simulink model "autopilot"  (R2020a)
settings: Solver=VariableStepAuto  StartTime=0.0  StopTime=10.0  RelTol=1e-3
values from neighbouring files (symbols this model uses):
  A = [-0.322, 0.052, 0.028, -1.12, 0.002 ... (first row only)    [main.m]
  B = [ (1-t_thr)  X_delta2 ... (first row only)    [Part1.m]    (also in main.m = [0; 0; 0; 0; 7.5;]; part2.m = 21.8; speed_control.m = 21.8)
  C = CRB + CA    [Part1.m]    (also in main.m = [1, 0,0,0,0)
  d = 1.5*pi/180    (= 0.0261799387799)    [main.m]    (also in part2.m = -[Xns Ycf Ncf]'; speed_control.m = -[Xns Ycf Ncf]')
  D = [0; 0; 0; 0;]    [main.m]    (also in part2.m = diag([-Xu -Yv -Nr]); problem4.m = [ Xu 0 0; speed_control.m = diag([-Xu -Yv -Nr]))
  g = 9.81    [main.m]
  kd_phi = (2*zeta_phi*omega_n_phi-a_phi_1)/a_phi_2    [main.m]
  ki_chi = omega_n_chi^2*V_g/g    [main.m]
  ki_phi = 0    [main.m]
  kp_chi = 2*zeta_chi*omega_n_chi*V_g/g    [main.m]
  kp_phi = delta_max/e_max*sign(a_phi_2)    [main.m]
  V_g = 580    [main.m]
libraries: simulink_extras x7
settings Model: Creator=erlended  LastModifiedBy=erlended

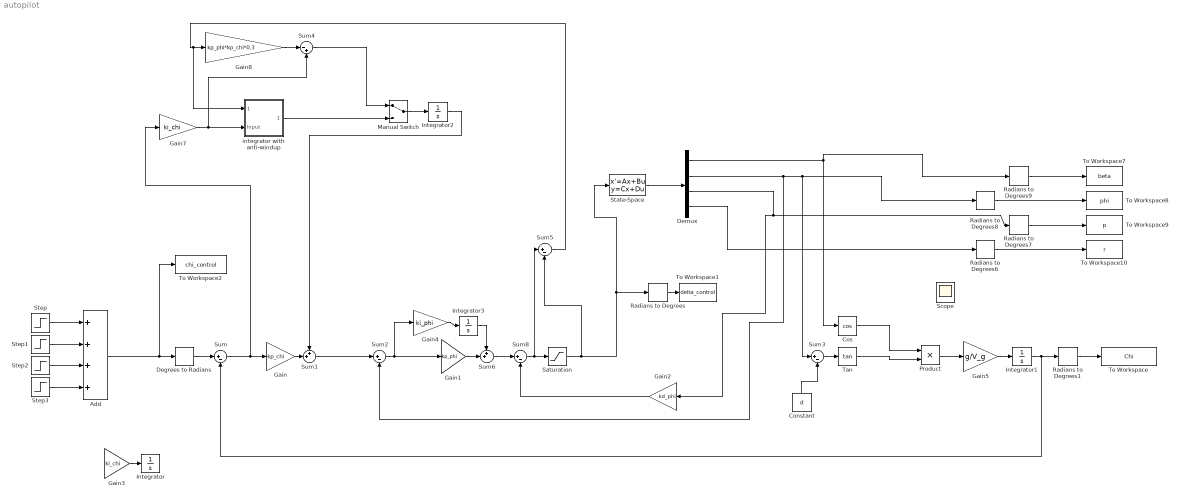
== system autopilot ==
  Add : Sum  Inputs=++++
  Constant : Constant  Value=d
  Cos : Trigonometry  Operator=cos
  Degrees to Radians : simulink_extras/Transformations/Degrees to Radians
  Demux : Demux
  Gain : Gain  Gain=kp_chi
  Gain1 : Gain  Gain=kp_phi
  Gain2 : Gain  Gain=kd_phi
  Gain3 : Gain  Gain=ki_chi
  Gain4 : Gain  Gain=ki_phi
  Gain5 : Gain  Gain=g/V_g
  Gain7 : Gain  Gain=ki_chi
  Gain8 : Gain  Gain=kp_phi*kp_chi*0.3
  Integrator{,1..3} (4 alike) : Integrator
  Manual Switch : ManualSwitch
  Product : Product
  Radians to Degrees{,1,6..9} (6 alike) : simulink_extras/Transformations/Radians to Degrees
  Saturation : Saturate  UpperLimit=pi/6  LowerLimit=-pi/6
  Scope : Scope
  State-Space : StateSpace  A=A  B=B  C=C  D=D  InitialCondition=0
  Step : Step  Time=100  After=7.5  SampleTime=0
  Step1 : Step  Time=150  After=7.5  SampleTime=0
  Step2 : Step  Time=250  After=-15  SampleTime=0
  Step3 : Step  Time=300  After=0  SampleTime=0
  Sum{,2..3,5,8} (5 alike) : Sum  Inputs=|+-
  Sum1 : Sum  Inputs=++|
  Sum4 : Sum  Inputs=|-+
  Sum6 : Sum  Inputs=++|
  Tan : Trigonometry  Operator=tan
  To Workspace : ToWorkspace  VariableName=Chi  SaveFormat=Timeseries  SampleTime=-1
  To Workspace1 : ToWorkspace  VariableName=delta_control  SaveFormat=Timeseries  SampleTime=-1
  To Workspace10 : ToWorkspace  VariableName=r  SaveFormat=Timeseries  SampleTime=-1
  To Workspace2 : ToWorkspace  VariableName=chi_control  SaveFormat=Timeseries  SampleTime=-1
  To Workspace7 : ToWorkspace  VariableName=beta  SaveFormat=Timeseries  SampleTime=-1
  To Workspace8 : ToWorkspace  VariableName=phi  SaveFormat=Timeseries  SampleTime=-1
  To Workspace9 : ToWorkspace  VariableName=p  SaveFormat=Timeseries  SampleTime=-1
  integrator with anti-windup : Subsystem
  wires:
  Sum/1 -> Gain7/1, Gain/1
  Gain/1 -> Sum1/2
  Sum1/1 -> Sum2/1
  Sum2/1 -> Gain1/1, Gain4/1
  Gain1/1 -> Sum6/2
  Integrator3/1 -> Sum6/1
  Gain2/1 -> Sum8/2
  Sum6/1 -> Sum8/1
  Sum8/1 -> Sum5/1, Saturation/1
  Integrator1/1 -> Radians to Degrees1/1, Sum/2
  Degrees to Radians/1 -> Sum/1
  Gain3/1 -> Integrator/1
  Gain4/1 -> Integrator3/1
  Product/1 -> Gain5/1
  Gain5/1 -> Integrator1/1
  Step1/1 -> Add/2
  Add/1 -> To Workspace2/1, Degrees to Radians/1
  Step/1 -> Add/1
  Step3/1 -> Add/4
  Step2/1 -> Add/3
  Radians to Degrees/1 -> To Workspace1/1
  Radians to Degrees1/1 -> To Workspace/1
  Saturation/1 -> State-Space/1, Radians to Degrees/1, Sum5/2
  Radians to Degrees6/1 -> To Workspace10/1
  Radians to Degrees8/1 -> To Workspace8/1
  Radians to Degrees9/1 -> To Workspace7/1
  Radians to Degrees7/1 -> To Workspace9/1
  Demux/1 -> Radians to Degrees9/1, Cos/1
  Tan/1 -> Product/2
  Cos/1 -> Product/1
  Demux/4 -> Radians to Degrees6/1
  Sum3/1 -> Tan/1
  Constant/1 -> Sum3/2
  Demux/2 -> Sum2/2, Radians to Degrees8/1, Sum3/1
  Demux/3 -> Gain2/1, Radians to Degrees7/1
  Gain8/1 -> Sum4/1
  integrator with anti-windup/1(Output) -> Manual Switch/2
  Sum4/1 -> Manual Switch/1
  Manual Switch/1 -> Integrator2/1
  Gain7/1 -> Sum4/2, integrator with anti-windup/2(Input)
  Integrator2/1 -> Sum1/1
  Sum5/1 -> integrator with anti-windup/1(delta_a), Gain8/1
  State-Space/1 -> Demux/1

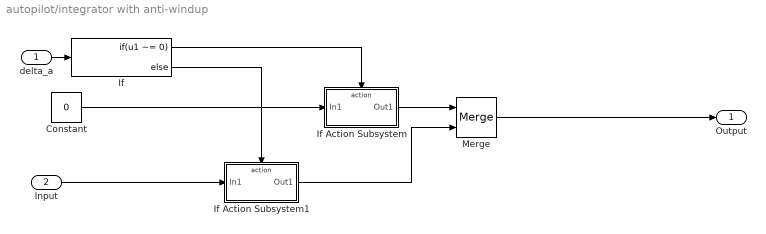
== system autopilot/integrator with anti-windup ==
  delta_a : Inport
  Input : Inport  Port=2
  Constant : Constant  Value=0
  If : If  IfExpression=u1 ~= 0
  If Action Subsystem : Subsystem  TreatAsAtomicUnit=on
  If Action Subsystem1 : Subsystem  TreatAsAtomicUnit=on
  Merge : Merge
  Output : Outport  VectorParamsAs1DForOutWhenUnconnected=off
  wires:
  If/2 -> If Action Subsystem1/Action
  If/1 -> If Action Subsystem/Action
  If Action Subsystem1/1(Out1) -> Merge/2
  If Action Subsystem/1(Out1) -> Merge/1
  delta_a/1 -> If/1
  Constant/1 -> If Action Subsystem/1(In1)
  Input/1 -> If Action Subsystem1/1(In1)
  Merge/1 -> Output/1

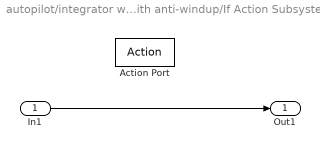
== system autopilot/integrator with anti-windup/If Action Subsystem ==
  In1 : Inport
  Action Port : ActionPort  ActionPortLabel=if(u1 ~= 0)
  Out1 : Outport  VectorParamsAs1DForOutWhenUnconnected=off
  wires:
  In1/1 -> Out1/1

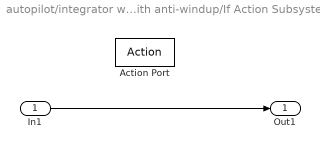
== system autopilot/integrator with anti-windup/If Action Subsystem1 ==
  In1 : Inport
  Action Port : ActionPort  ActionPortLabel=else
  Out1 : Outport  VectorParamsAs1DForOutWhenUnconnected=off
  wires:
  In1/1 -> Out1/1
